simulink model "mophonghexe"  (R2019a)
settings: Solver=VariableStepAuto  StartTime=0.0  StopTime=10  RelTol=1e-3
values from neighbouring files (symbols this model uses):
  A = (m1*l1 + m2*l2)*g / D    (= 6.125)    [init_xe.m]
  As = (m1s*l1s + m2s*l2s)*g / Ds    [init_xe.m]
  B = -1 / D    (= -0.125)    [init_xe.m]
  Ds = m1s*(l1s^2) + m2s*(l2s^2) + I1s    [init_xe.m]
  I2 = 1    [init_xe.m]
libraries: simulink x3
settings Model: Creator=khoa  LastModifiedBy=Ly Kien
settings DataIOCC: ReturnWorkspaceOutputs=off
settings OptimizationCC: DefaultUnderspecifiedDataType=single
settings DebuggingCC: PregeneratedLibrarySubsystemCodeDiagnostic=none  ArithmeticOperatorsInVariantConditions=warning
settings SFSimCC: SimUseLocalCustomCode=off
settings RTWCC: RTWUseLocalCustomCode=off

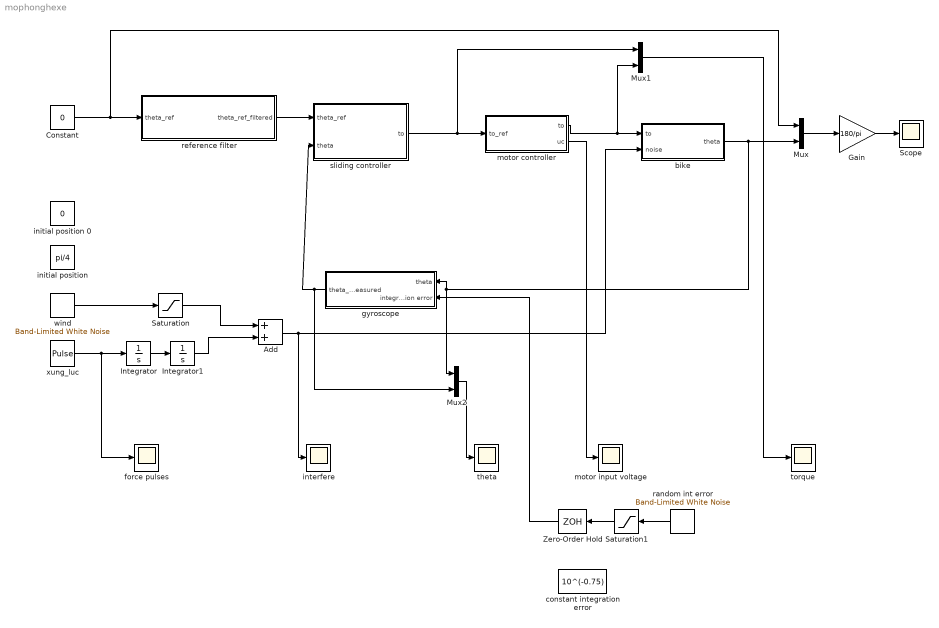
== system mophonghexe ==
  Add : Sum
  Constant : Constant  Value=0
  Gain : Gain  Gain=180/pi
  Integrator : Integrator
  Integrator1 : Integrator
  Mux : Mux  Inputs=2
  Mux1 : Mux  Inputs=2
  Mux2 : Mux  Inputs=2
  Saturation : Saturate  UpperLimit=pi/36  LowerLimit=-pi/36
  Saturation1 : Saturate  UpperLimit=pi/72  LowerLimit=-pi/72
  Scope : Scope
  Zero-Order Hold : ZeroOrderHold  SampleTime=0.002
  bike : Subsystem
  constant integration error : Constant  Value=10^(-0.75)
  force pulses : Scope
  gyroscope : Subsystem
  initial position : Constant  Value=pi/4
  initial position 0 : Constant  Value=0
  interfere : Scope
  motor controller : Subsystem
  motor input voltage : Scope
  random int error : simulink/Sources/Band-Limited White Noise  Cov=[(pi^2)/(128^2)]  Ts=0.002  seed=[133248]
  reference filter : Subsystem
  sliding controller : Subsystem
  theta : Scope
  torque : Scope
  wind : simulink/Sources/Band-Limited White Noise  Cov=[(pi^2)/(72^2)]  Ts=0.1  seed=[23341]
  "xung_luc " : DiscretePulseGenerator  PulseType=Time based  Amplitude=420  Period=4  PulseWidth=10  PhaseDelay=1
  wires:
  sliding controller/1(to) -> Mux1/1, motor controller/1(to_ref)
  Constant/1 -> reference filter/1(theta_ref), Mux/1
  wind/1 -> Saturation/1
  motor controller/1(to) -> Mux1/2, bike/1(to)
  Mux/1 -> Gain/1
  Mux1/1 -> torque/1
  Add/1 -> interfere/1, bike/2(noise)
  "xung_luc "/1 -> force pulses/1, Integrator/1
  Integrator/1 -> Integrator1/1
  Saturation/1 -> Add/1
  Integrator1/1 -> Add/2
  reference filter/1(theta_ref_filtered) -> sliding controller/1(theta_ref)
  Gain/1 -> Scope/1
  motor controller/2(uc) -> motor input voltage/1
  bike/1(theta) -> Mux2/1, gyroscope/1(theta), Mux/2
  gyroscope/1(theta_measured) -> Mux2/2, sliding controller/2(theta)
  Mux2/1 -> theta/1
  random int error/1 -> Saturation1/1
  Saturation1/1 -> Zero-Order Hold/1
  Zero-Order Hold/1 -> gyroscope/2(integration error)

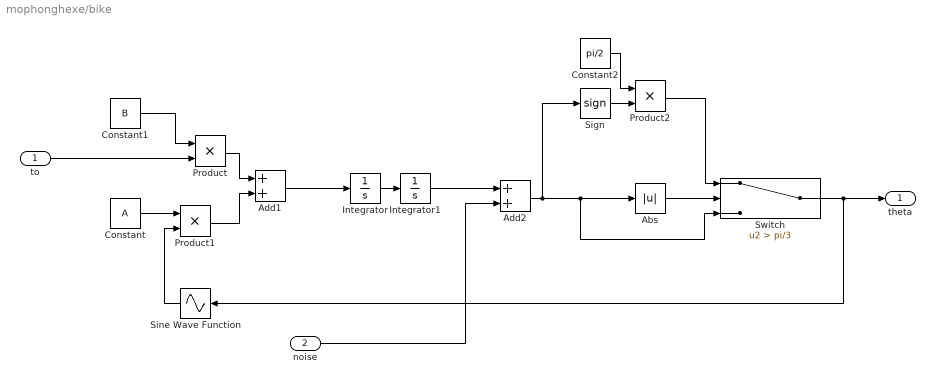
== system mophonghexe/bike ==
  to : Inport  PortDimensions=1
  noise : Inport  Port=2  PortDimensions=1
  Abs : Abs
  Add1 : Sum
  Add2 : Sum
  Constant : Constant  Value=A
  Constant1 : Constant  Value=B
  Constant2 : Constant  Value=pi/2
  Integrator : Integrator
  Integrator1 : Integrator
  Product : Product
  Product1 : Product
  Product2 : Product
  Sign : Signum
  Sine Wave Function : Sin  TimeSource=Use external signal  SampleTime=0
  Switch : Switch  Criteria=u2 > Threshold  Threshold=pi/3
  theta : Outport  PortDimensions=1
  wires:
  Integrator/1 -> Integrator1/1
  to/1 -> Product/2
  Product/1 -> Add1/1
  Product1/1 -> Add1/2
  Add1/1 -> Integrator/1
  Constant1/1 -> Product/1
  Constant/1 -> Product1/1
  Sine Wave Function/1 -> Product1/2
  Integrator1/1 -> Add2/1
  noise/1 -> Add2/2
  Add2/1 -> Abs/1, Switch/3, Sign/1
  Abs/1 -> Switch/2
  Sign/1 -> Product2/2
  Constant2/1 -> Product2/1
  Product2/1 -> Switch/1
  Switch/1 -> Sine Wave Function/1, theta/1

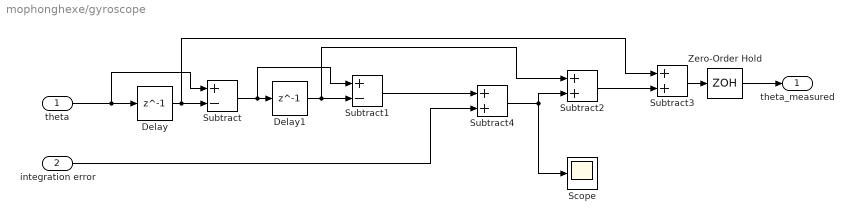
== system mophonghexe/gyroscope ==
  theta : Inport
  integration error : Inport  Port=2
  Delay : Delay  DelayLength=1  InitialCondition=0  SampleTime=0.002
  Delay1 : Delay  DelayLength=1  InitialCondition=0  SampleTime=0.002
  Scope : Scope
  Subtract : Sum  Inputs=+-
  Subtract1 : Sum  Inputs=+-
  Subtract2 : Sum
  Subtract3 : Sum
  Subtract4 : Sum
  Zero-Order Hold : ZeroOrderHold  SampleTime=-1
  theta_measured : Outport
  wires:
  theta/1 -> Subtract/1, Delay/1
  Delay/1 -> Subtract/2, Subtract3/1
  Subtract/1 -> Subtract1/1, Delay1/1
  Delay1/1 -> Subtract2/1, Subtract1/2
  Subtract2/1 -> Subtract3/2
  Subtract3/1 -> Zero-Order Hold/1
  Zero-Order Hold/1 -> theta_measured/1
  Subtract1/1 -> Subtract4/1
  Subtract4/1 -> Scope/1, Subtract2/2
  integration error/1 -> Subtract4/2

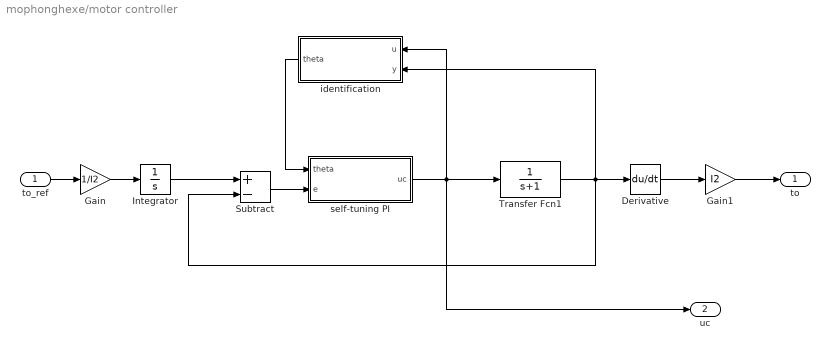
== system mophonghexe/motor controller ==
  to_ref : Inport
  Derivative : Derivative
  Gain : Gain  Gain=1/I2
  Gain1 : Gain  Gain=I2
  Integrator : Integrator
  Subtract : Sum  Inputs=+-
  Transfer Fcn1 : TransferFcn  Denominator=[1 1]
  identification : Subsystem
  self-tuning PI : Subsystem
  to : Outport
  uc : Outport  Port=2
  wires:
  to_ref/1 -> Gain/1
  identification/1(theta) -> self-tuning PI/1(theta)
  Subtract/1 -> self-tuning PI/2(e)
  self-tuning PI/1(uc) -> Transfer Fcn1/1, identification/1(u), uc/1
  Transfer Fcn1/1 -> Derivative/1, identification/2(y), Subtract/2
  Gain/1 -> Integrator/1
  Integrator/1 -> Subtract/1
  Derivative/1 -> Gain1/1
  Gain1/1 -> to/1

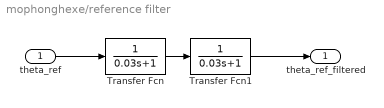
== system mophonghexe/reference filter ==
  theta_ref : Inport
  Transfer Fcn : TransferFcn  Denominator=[0.03 1]
  Transfer Fcn1 : TransferFcn  Denominator=[0.03 1]
  theta_ref_filtered : Outport
  wires:
  Transfer Fcn/1 -> Transfer Fcn1/1
  theta_ref/1 -> Transfer Fcn/1
  Transfer Fcn1/1 -> theta_ref_filtered/1

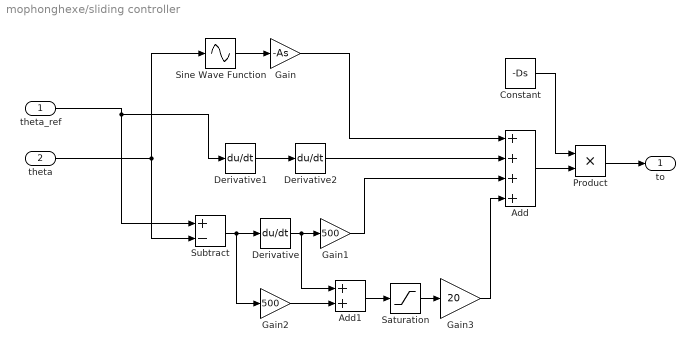
== system mophonghexe/sliding controller ==
  theta_ref : Inport
  theta : Inport  Port=2
  Add : Sum  Inputs=++++
  Add1 : Sum
  Constant : Constant  Value=-Ds
  Derivative : Derivative
  Derivative1 : Derivative
  Derivative2 : Derivative
  Gain : Gain  Gain=-As
  Gain1 : Gain  Gain=500
  Gain2 : Gain  Gain=500
  Gain3 : Gain  Gain=20
  Product : Product
  Saturation : Saturate  UpperLimit=20  LowerLimit=-20
  Sine Wave Function : Sin  TimeSource=Use external signal  SampleTime=0
  Subtract : Sum  Inputs=+-
  to : Outport
  wires:
  theta_ref/1 -> Derivative1/1, Subtract/1
  theta/1 -> Sine Wave Function/1, Subtract/2
  Sine Wave Function/1 -> Gain/1
  Gain/1 -> Add/1
  Subtract/1 -> Gain2/1, Derivative/1
  Gain1/1 -> Add/3
  Derivative/1 -> Add1/1, Gain1/1
  Gain2/1 -> Add1/2
  Add1/1 -> Saturation/1
  Saturation/1 -> Gain3/1
  Add/1 -> Product/2
  Constant/1 -> Product/1
  Product/1 -> to/1
  Gain3/1 -> Add/4
  Derivative1/1 -> Derivative2/1
  Derivative2/1 -> Add/2

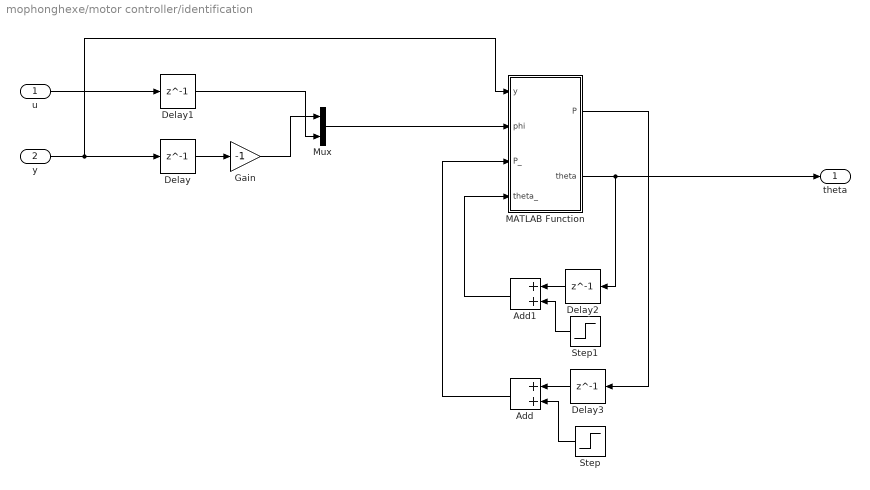
== system mophonghexe/motor controller/identification ==
  u : Inport  PortDimensions=1
  y : Inport  Port=2  PortDimensions=1
  Add : Sum
  Add1 : Sum
  Delay{,1..3} (4 alike) : Delay  DelayLength=1  InitialCondition=0  SampleTime=0.002
  Gain : Gain  Gain=-1
  MATLAB Function : MATLAB Function  TreatAsAtomicUnit=on
  Mux : Mux  Inputs=2
  Step : Step  Time=0.002  Before=eye(2)  After=zeros(2)  SampleTime=0
  Step1 : Step  Time=0.002  Before=[1 1]'  After=[0 0]'  SampleTime=0
  theta : Outport  PortDimensions=2
  wires:
  y/1 -> MATLAB Function/1(y), Delay/1
  u/1 -> Delay1/1
  Delay/1 -> Gain/1
  Gain/1 -> Mux/1
  Delay1/1 -> Mux/2
  Mux/1 -> MATLAB Function/2(phi)
  MATLAB Function/2(theta) -> theta/1, Delay2/1
  Step/1 -> Add/2
  MATLAB Function/1(P) -> Delay3/1
  Step1/1 -> Add1/2
  Add1/1 -> MATLAB Function/4(theta_)
  Add/1 -> MATLAB Function/3(P_)
  Delay2/1 -> Add1/1
  Delay3/1 -> Add/1

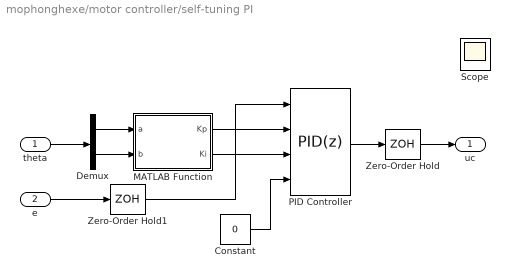
== system mophonghexe/motor controller/self-tuning PI ==
  theta : Inport  PortDimensions=2
  e : Inport  Port=2  PortDimensions=1
  Constant : Constant  Value=0
  Demux : Demux  Outputs=2
  MATLAB Function : MATLAB Function  TreatAsAtomicUnit=on
  PID Controller : simulink/Continuous/PID Controller  Controller=PID  Form=Parallel  TimeDomain=Discrete-time  SampleTime=0.002  IntegratorMethod=Trapezoidal  FilterMethod=Forward Euler  ControllerParametersSource=external  P=753.7538  I=605.6056  D=0  UseFilter=off  N=100  TunerSelectOption=Transfer Function Based (PID Tuner App)  InitialConditionSource=internal  InitialConditionForIntegrator=0  InitialConditionForFilter=0  DifferentiatorICPrevScaledInput=0  ExternalReset=none  TrackingMode=off  Kt=1  LimitOutput=off  UpperSaturationLimit=inf  LowerSaturationLimit=-inf  LinearizeAsGain=on  AntiWindupMode=none  Kb=1  POutMin=[]  POutMax=[]  IOutMin=[]  IOutMax=[]  DOutMin=[]  DOutMax=[]  NOutMin=[]  NOutMax=[]  SumOutMin=[]  SumOutMax=[]  SaturationOutMin=[]  SaturationOutMax=[]  PParamMin=[]  PParamMax=[]  IParamMin=[]  IParamMax=[]  DParamMin=[]  DParamMax=[]  NParamMin=[]  NParamMax=[]  KbParamMin=[]  KbParamMax=[]  KtParamMin=[]  KtParamMax=[]  KbOutMin=[]  KbOutMax=[]  KtOutMin=[]  KtOutMax=[]  IntegratorOutMin=[]  IntegratorOutMax=[]  FilterOutMin=[]  FilterOutMax=[]  SumI1OutMin=[]  SumI1OutMax=[]  SumI2OutMin=[]  SumI2OutMax=[]  SumI3OutMin=[]  SumI3OutMax=[]  SumI4OutMin=[]  SumI4OutMax=[]  SumDOutMin=[]  SumDOutMax=[]  DifferentiatorOutMin=[]  DifferentiatorOutMax=[]  FilterDiffOutCoefMin=[]  FilterDiffOutCoefMax=[]  ReciprocalOutMin=[]  ReciprocalOutMax=[]  SumDenOutMin=[]  SumDenOutMax=[]  SumNumOutMin=[]  SumNumOutMax=[]  DivideOutMin=[]  DivideOutMax=[]  IntegratorContinuousStateAttributes=''  IntegratorStateMustResolveToSignalObject=off  IntegratorRTWStateStorageClass=Auto  FilterContinuousStateAttributes=''  FilterStateMustResolveToSignalObject=off  FilterRTWStateStorageClass=Auto  ParallelPVariant=ExternalParameters  IdealPVariant=Disabled  IVariant=ExternalParameters  DVariant=ExternalParameters  IntegratorVariant=Discrete  SatVariant=Disabled  AWVariant=Passthrough  PCopyVariant=Disabled  TRVariant=Disabled  FdbkBlocksVariant=Forward  IdealPFdbkVariant=Disabled  SatFdbkVariant=Disabled  DerivativeFilterVariant=Differentiator  NVariant=Passthrough  NCopyVariant=Disabled_SignalSpec  FilterICVariant=InternalICsDifferentiator  IntegratorICVariant=InternalICs  ExternalResetVariant=Disabled  TRSumVariant=Passthrough  SumFdbkVariant=Disabled  SumVariant=Sum_PID
  Scope : Scope
  Zero-Order Hold : ZeroOrderHold  SampleTime=-1
  Zero-Order Hold1 : ZeroOrderHold  SampleTime=0.002
  uc : Outport  PortDimensions=1
  wires:
  Constant/1 -> PID Controller/4
  e/1 -> Zero-Order Hold1/1
  MATLAB Function/1(Kp) -> PID Controller/2
  MATLAB Function/2(Ki) -> PID Controller/3
  Demux/1 -> MATLAB Function/1(a)
  Demux/2 -> MATLAB Function/2(b)
  theta/1 -> Demux/1
  PID Controller/1 -> Zero-Order Hold/1
  Zero-Order Hold/1 -> uc/1
  Zero-Order Hold1/1 -> PID Controller/1

== matlab function mophonghexe/motor controller/identification/MATLAB Function ==
  data: y input; P output; phi input; P_ input; theta_ input; theta output
function [P, theta] = fcn(y, phi, P_, theta_)

lambda = 0.998;

P = (1/lambda) * (P_ - (P_*phi*(phi')*P_)/(lambda + (phi')*P_*phi));
L = (P_*phi)/(lambda + (phi')*P_*phi);
epsilon = y - phi'*theta_;

theta = theta_ + L*epsilon;

end

== matlab function mophonghexe/motor controller/self-tuning PI/MATLAB Function ==
  data: a input; Kp output; b input; Ki output
function [Kp, Ki] = fcn(a, b)

Kp = 1.21/b;
Ki = (0.508-a)/b;

end
